simulink model "Y_Model"  (R2017a)
settings: Solver=VariableStepAuto  StartTime=0.0  StopTime=sim_time  RelTol=1e-3
values from neighbouring files (symbols this model uses):
  D_Model_SISO = cell(6,1)    [DigitalControlsProject1.m]
  K_test = cell(6,1)    [DigitalControlsProject1.m]
  N = cell(6,1)    [DigitalControlsProject1.m]
  T = 1/40    (= 0.025)    [DigitalControlsProject1.m]
settings Model: Creator=Alphakyl  LastModifiedBy=windo

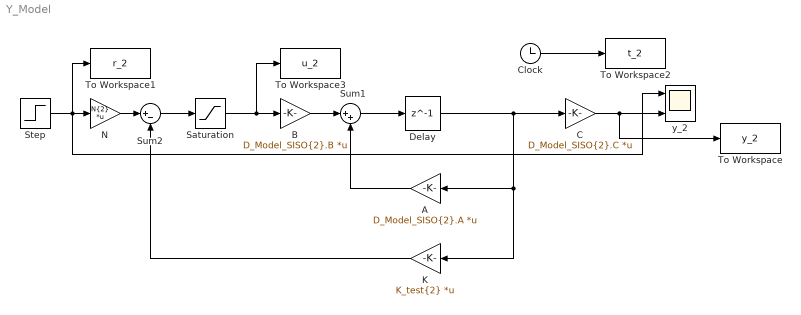
== system Y_Model ==
  A : Gain  Gain=D_Model_SISO{2}.A  Multiplication=Matrix(K*u)
  B : Gain  Gain=D_Model_SISO{2}.B  Multiplication=Matrix(K*u)
  C : Gain  Gain=D_Model_SISO{2}.C  Multiplication=Matrix(K*u)
  Clock : Clock
  Delay : Delay  DelayLength=1  SampleTime=T
  K : Gain  Gain=K_test{2}  Multiplication=Matrix(K*u)
  N : Gain  Gain=N{2}  Multiplication=Matrix(K*u)
  Saturation : Saturate  UpperLimit=100  LowerLimit=-100
  Step : Step  SampleTime=T
  Sum1 : Sum  Inputs=|++
  Sum2 : Sum  Inputs=|+-
  To Workspace : ToWorkspace  VariableName=y_2  SampleTime=-1
  To Workspace1 : ToWorkspace  VariableName=r_2  SampleTime=-1
  To Workspace2 : ToWorkspace  VariableName=t_2  SampleTime=-1
  To Workspace3 : ToWorkspace  VariableName=u_2  SampleTime=-1
  y_2 : Scope  NumInputPorts=2
  wires:
  C/1 -> To Workspace/1, y_2/2
  N/1 -> Sum2/1
  Step/1 -> To Workspace1/1, y_2/1, N/1
  B/1 -> Sum1/1
  Delay/1 -> A/1, K/1, C/1
  Sum2/1 -> Saturation/1
  K/1 -> Sum2/2
  A/1 -> Sum1/2
  Sum1/1 -> Delay/1
  Clock/1 -> To Workspace2/1
  Saturation/1 -> To Workspace3/1, B/1
